simulink model "Mimo_non_linear_control"  (R2024b)
settings: Solver=FixedStepAuto  StartTime=0.0  StopTime=20  FixedStep=0.00001  RelTol=1e-3
settings Model: Creator=olive  LastModifiedBy=olive

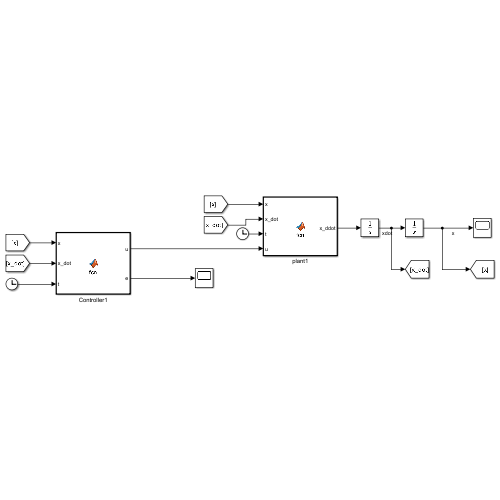
[thumbnail: Simulink's stored preview of the top-level diagram]
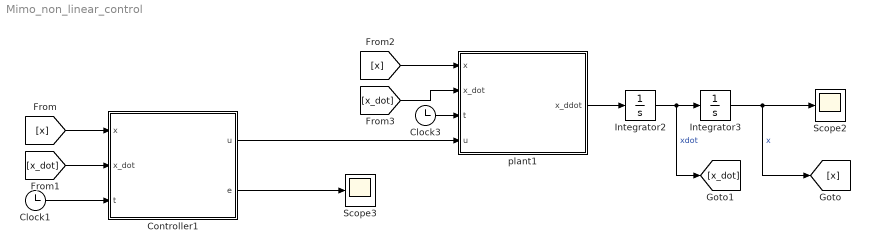
== system Mimo_non_linear_control ==
  Clock1 : Clock
  Clock3 : Clock
  Controller1 : MATLAB Function  TreatAsAtomicUnit=on
  Integrator2 : Integrator  InitialCondition=[0;0]
  Integrator3 : Integrator  InitialCondition=[0;0]
  Scope2 : Scope
  Scope3 : Scope
  plant1 : MATLAB Function  TreatAsAtomicUnit=on
  wires:
  Clock1/1 -> Controller1/3(t)
  [x] -> plant1/1(x)
  [x_dot] -> plant1/2(x_dot)
  [x] -> Controller1/1(x)
  Controller1/2(e) -> Scope3/1
  Integrator2/1 -> [x_dot], Integrator3/1  "xdot"
  [x_dot] -> Controller1/2(x_dot)
  Controller1/1(u) -> plant1/4(u)
  plant1/1(x_ddot) -> Integrator2/1
  Integrator3/1 -> [x], Scope2/1  "x"
  Clock3/1 -> plant1/3(t)

== matlab function Mimo_non_linear_control/Controller1 ==
  settings: updateMethod=DISCRETE
  data: x input; u output; x_dot input; t input; e output
function [u,e] = fcn(x,x_dot,t)
%defining f&g
f = [sin(x_dot(2))*x(1)+cos(t)*x(2);
    10*x_dot(1)+sin(t)*sin(t)*x(2)*x_dot(1)];
g = [2 0;
     0 1];
% defining R
r = [10 + sin(0.1*t);
     5 + cos(2*t)];
r_dot = [0.1*cos(0.1*t);
        -2*sin(2*t)];
r_ddot = [-0.01*sin(0.1*t);
          -4*cos(2*t)];
e = x-r;
e_dot = x_dot - r_dot;

kp = 10;
kd = 1;

u = (g^(-1))*(- f - kp*e - kd*e_dot + r_ddot);
end

== matlab function Mimo_non_linear_control/plant1 ==
  settings: updateMethod=DISCRETE
  data: x input; x_dot input; t input; u input; x_ddot output
function x_ddot = fcn(x,x_dot,t,u)
%defining f&g
f = [sin(x_dot(2))*x(1)+cos(t)*x(2);
    10*x_dot(1)+sin(t)*sin(t)*x(2)*x_dot(1)];
g = [2 0;
     0 1];

x_ddot = f + g*u;
end
